simulink model "dr_district_workflow_basic"  (R2026a)
settings: Solver=FixedStepDiscrete  StopTime=1500  FixedStep=1
model workspace (MAT data in the model file):
  cfg.opts.mdl = 'dr_district_workflow_basic'
  cfg.opts.patientsPerYear = 100000
  cfg.opts.workingDaysPerYear = 250
  cfg.opts.hoursPerDay = 6
  cfg.opts.nOphthalmologists = 8
  cfg.opts.aiEnabled = 0
  cfg.opts.maxRecaptures = 2
  cfg.opts.paramFile = 'measured_params.json'
  cfg.params.generated_at = '2026-09-11T16:26:06.379668+00:00'
  cfg.params.source = 'MEASURED: service times from live API traffic; rates from 80 held-out APTOS validation images through the full pipeline (model aptos-kaggle-run1)'
  cfg.params.n_scans = 6
  cfg.params.qualityGateSeconds = 0.05
  cfg.params.gradingSeconds = 3.017
  cfg.params.ungradeableRate = 0
  cfg.params.reviewSeconds = 18.2
  cfg.params.uploadSeconds = 5.5
  cfg.params.uploadSeconds_basis = '350 kB downscaled JPEG over a 512 kbit/s rural link'
  cfg.params.recaptureSeconds = 45
  cfg.params.recaptureSeconds_basis = 'assumption: health worker repositions and retakes'
  cfg.params.referableRate = 0.4
  cfg.params.NOTE = 'needsHumanRate (0.725) is MEASURED directly as ''referable OR escalated to clinician'', de-duplicated. Do NOT sum referableRate and disagreementRate: an image can be both, and summing gives 1.14 which is impossible. ungradeableRate is 0.0 because the quality thresholds, fitted on 13 synthetic images, refuse essentially no real APTOS image (1 of 550 val, 0 of 400 test). That is a known defect, not a property of the data.'
  cfg.params.rates_measured_at = '2026-09-13T15:50:04.983407Z'
  cfg.params.rates_n = 80
  cfg.params.needsHumanRate = 0.725
  cfg.params.flag_breakdown.agree = 21
  cfg.params.flag_breakdown.severity_disagreement = 19
  cfg.params.flag_breakdown.referral_disagreement = 33
  cfg.params.flag_breakdown.rules_cannot_confirm = 7
  cfg.params.unmeasured_fields = {'manualReadSeconds'}
  cfg.params.manualReadSeconds = 120
  cfg.arrivalsPerHr = 66.6666666667
  cfg.capacityPerHr = 240
  cfg.needsHumanFrac = 1
  cfg.gradeableFrac = 1
  cfg.secondsPerRead = 120
undefined symbols (not defined in the file or in its folder): DiscIntNeverNeededParam
settings Model: Creator=ganesh  LastModifiedBy=ganesh

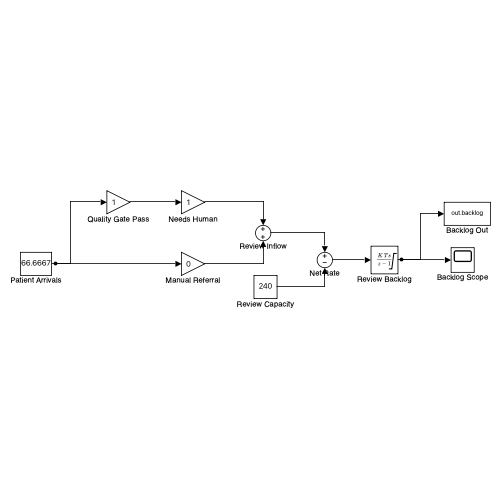
[thumbnail: Simulink's stored preview of the top-level diagram]
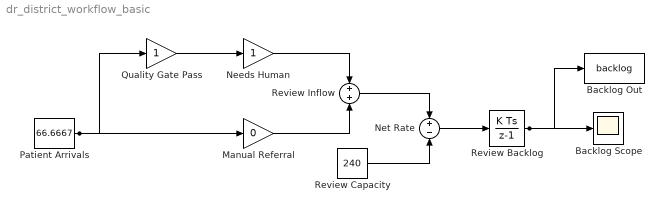
== system dr_district_workflow_basic ==
  Backlog Out : ToWorkspace  VariableName=backlog  SaveFormat=Timeseries  SampleTime=-1
  Backlog Scope : Scope
  Manual Referral : Gain  Gain=0
  Needs Human : Gain
  Net Rate : Sum  Inputs=+-
  Patient Arrivals : Constant  Value=66.6667  SampleTime=1
  Quality Gate Pass : Gain
  Review Backlog : DiscreteIntegrator  LimitOutput=on  LowerSaturationLimit=0  ICPrevOutput=DiscIntNeverNeededParam  ICPrevScaledInput=DiscIntNeverNeededParam
  Review Capacity : Constant  Value=240  SampleTime=1
  Review Inflow : Sum
  wires:
  Review Backlog/1 -> Backlog Scope/1, Backlog Out/1
  Net Rate/1 -> Review Backlog/1
  Review Capacity/1 -> Net Rate/2
  Patient Arrivals/1 -> Quality Gate Pass/1, Manual Referral/1
  Needs Human/1 -> Review Inflow/1
  Review Inflow/1 -> Net Rate/1
  Manual Referral/1 -> Review Inflow/2
  Quality Gate Pass/1 -> Needs Human/1
